simulink subsystem "ControladorBA"  (R2023b)
settings: Solver=VariableStepAuto  StartTime=0.0  StopTime=10.0  RelTol=1e-3
settings Model: Creator=johan  LastModifiedBy=adria

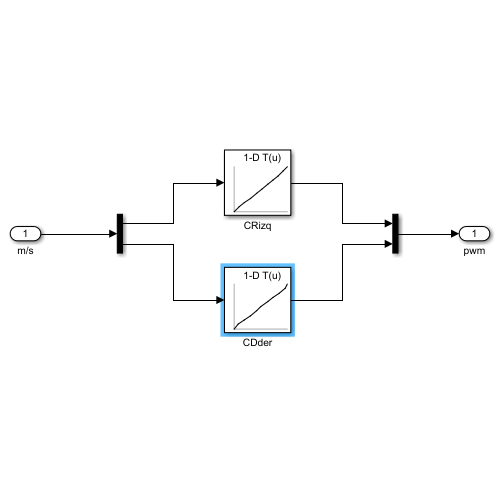
[thumbnail: Simulink's stored preview of the top-level diagram]
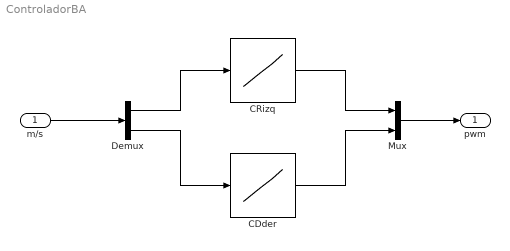
== system ControladorBA ==
  m/s : Inport
  CDder : Lookup_n-D  NumberOfTableDimensions=1  BreakpointsForDimension1=[-0.334034651517868 -0.276784002780914 -0.200431555509567 -0.133619040250778 -0.057269562035799 0 0.085894286632538 0.15270359814167 0.219512194395065 0.305411517620087 0.324499905109406]  Table=[-255 -200 -150 -100 -50 0 50 100 150 200 255]  InternalRulePriority=Speed  RndMeth=Simplest
  CRizq : Lookup_n-D  NumberOfTableDimensions=1  BreakpointsForDimension1=[-0.52526581287384 -0.414703637361527 -0.317939072847366 -0.207345858216286 -0.096764579415321 0 0.124403968453407 0.221168518066406 0.331753820180893 0.414687782526016 0.497627735137939]  Table=[-255 -200 -150 -100 -50 0 50 100 150 200 255]  InternalRulePriority=Speed  RndMeth=Simplest
  Demux : Demux  Outputs=2
  Mux : Mux  Inputs=2
  pwm : Outport
  wires:
  CDder/1 -> Mux/2
  m/s/1 -> Demux/1
  Mux/1 -> pwm/1
  Demux/1 -> CRizq/1
  Demux/2 -> CDder/1
  CRizq/1 -> Mux/1
